simulink model "MovingAvg3"  (R2024b)
settings: Solver=FixedStepAuto  StartTime=0.0  StopTime=1500  FixedStep=1/3600  RelTol=1e-3
undefined symbols (not defined in the file or in its folder): sigbuilder_block
libraries: dspspect3 x1
settings Model: SimulationMode=accelerator  Creator=rupak  LastModifiedBy=rupak
settings ModelReferenceCC: EnableRefExpFcnMdlSchedulingChecks=on
settings RTWCC: GPUComputeCapability=3.5
settings ConfigComp: DVTestSuiteOptimization=Auto  DVDefectChecker=off  DVDetectOutOfBounds=on  DVModelReferenceHarness=on  DVHarnessSource=Signal Editor

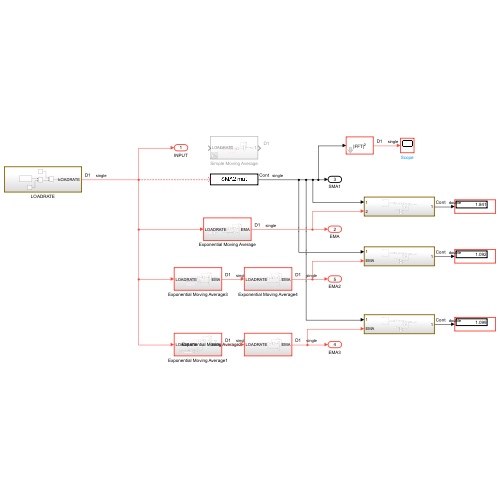
[thumbnail: Simulink's stored preview of the top-level diagram]
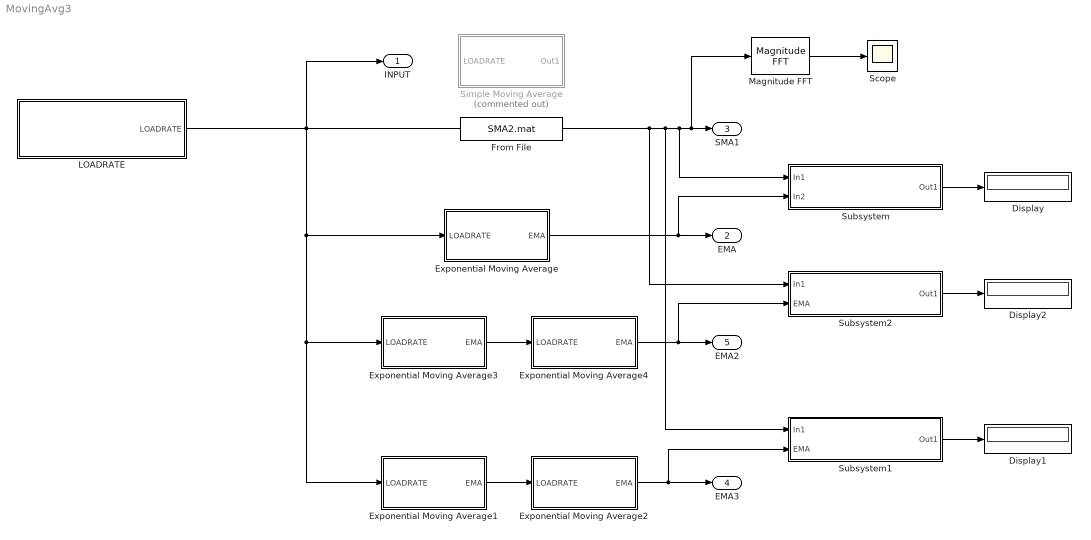
== system MovingAvg3 ==
  Display : Display
  Display1 : Display
  Display2 : Display
  Exponential Moving Average : Subsystem
  Exponential Moving Average1 : Subsystem
  Exponential Moving Average2 : Subsystem
  Exponential Moving Average3 : Subsystem
  Exponential Moving Average4 : Subsystem
  From File : FromFile  FileName=SMA2.mat  SampleTime=0
  LOADRATE : Subsystem
  Magnitude FFT : dspspect3/Magnitude FFT  mag_or_magsq=Magnitude squared  FFTImplementation=Auto  fftLenInherit=off  fftsize=256  WrapInput=on
      settings: LibrarySourceBlock=|
      | dspxfrm3/Magnitude
      | FFT
  Scope : Scope
  Simple Moving Average : Subsystem  Commented=on
  Subsystem : Subsystem
  Subsystem1 : Subsystem
  Subsystem2 : Subsystem
  INPUT : Outport
  EMA : Outport  Port=2
  SMA1 : Outport  Port=3
  EMA3 : Outport  Port=4
  EMA2 : Outport  Port=5
  wires:
  Exponential Moving Average/1(EMA) -> EMA/1, Subsystem/2(In2)
  From File/1 -> Subsystem2/1(In1), Subsystem1/1(In1), Subsystem/1(In1), Magnitude FFT/1, SMA1/1
  Exponential Moving Average1/1(EMA) -> Exponential Moving Average2/1(LOADRATE)
  Exponential Moving Average2/1(EMA) -> EMA3/1, Subsystem1/2(EMA)
  LOADRATE/1(LOADRATE) -> Exponential Moving Average3/1(LOADRATE), Exponential Moving Average1/1(LOADRATE), Exponential Moving Average/1(LOADRATE), INPUT/1
  Subsystem/1(Out1) -> Display/1
  Subsystem1/1(Out1) -> Display1/1
  Exponential Moving Average3/1(EMA) -> Exponential Moving Average4/1(LOADRATE)
  Exponential Moving Average4/1(EMA) -> Subsystem2/2(EMA), EMA2/1
  Subsystem2/1(Out1) -> Display2/1
  Magnitude FFT/1 -> Scope/1

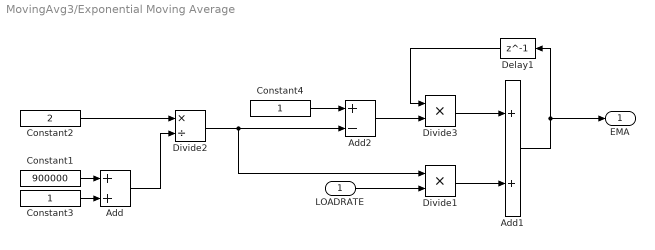
== system MovingAvg3/Exponential Moving Average ==
  LOADRATE : Inport
  Add : Sum
  Add1 : Sum
  Add2 : Sum  Inputs=+-
  Constant1 : Constant  Value=900000  OutDataTypeStr=single
  Constant2 : Constant  Value=2  OutDataTypeStr=single
  Constant3 : Constant  OutDataTypeStr=single
  Constant4 : Constant  OutDataTypeStr=single
  Delay1 : Delay  DelayLength=1  InitialCondition=60
  Divide1 : Product  Inputs=**
  Divide2 : Product  Inputs=*/
  Divide3 : Product  Inputs=**
  EMA : Outport
  wires:
  Add1/1 -> EMA/1, Delay1/1
  Divide1/1 -> Add1/2
  Constant2/1 -> Divide2/1
  Constant1/1 -> Add/1
  Constant3/1 -> Add/2
  Add/1 -> Divide2/2
  Delay1/1 -> Divide3/1
  Divide3/1 -> Add1/1
  Add2/1 -> Divide3/2
  Constant4/1 -> Add2/1
  Divide2/1 -> Add2/2, Divide1/1
  LOADRATE/1 -> Divide1/2

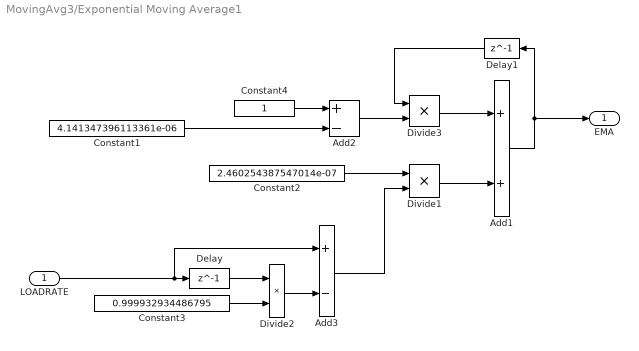
== system MovingAvg3/Exponential Moving Average1 ==
  LOADRATE : Inport
  Add1 : Sum
  Add2 : Sum  Inputs=+-
  Add3 : Sum  Inputs=+-
  Constant1 : Constant  Value=4.141347396113361e-06  OutDataTypeStr=single
  Constant2 : Constant  Value=2.460254387547014e-07  OutDataTypeStr=single
  Constant3 : Constant  Value=0.999932934486795  OutDataTypeStr=single
  Constant4 : Constant  OutDataTypeStr=single
  Delay : Delay  DelayLength=1  InitialCondition=60
  Delay1 : Delay  DelayLength=1  InitialCondition=0.000238234
  Divide1 : Product  Inputs=**
  Divide2 : Product  Inputs=**
  Divide3 : Product  Inputs=**
  EMA : Outport
  wires:
  Add1/1 -> EMA/1, Delay1/1
  Divide1/1 -> Add1/2
  Delay1/1 -> Divide3/1
  Divide3/1 -> Add1/1
  Add2/1 -> Divide3/2
  Constant4/1 -> Add2/1
  Constant1/1 -> Add2/2
  LOADRATE/1 -> Add3/1, Delay/1
  Delay/1 -> Divide2/1
  Constant3/1 -> Divide2/2
  Add3/1 -> Divide1/2
  Divide2/1 -> Add3/2
  Constant2/1 -> Divide1/1

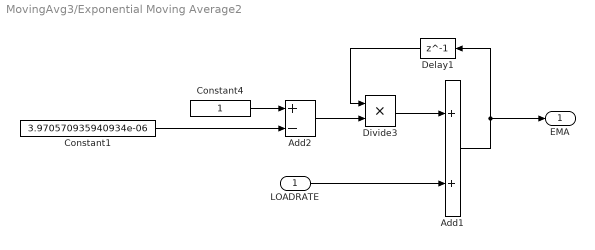
== system MovingAvg3/Exponential Moving Average2 ==
  LOADRATE : Inport
  Add1 : Sum
  Add2 : Sum  Inputs=+-
  Constant1 : Constant  Value=3.970570935940934e-06  OutDataTypeStr=single
  Constant4 : Constant  OutDataTypeStr=single
  Delay1 : Delay  DelayLength=1  InitialCondition=60
  Divide3 : Product  Inputs=**
  EMA : Outport
  wires:
  Add1/1 -> EMA/1, Delay1/1
  LOADRATE/1 -> Add1/2
  Delay1/1 -> Divide3/1
  Divide3/1 -> Add1/1
  Add2/1 -> Divide3/2
  Constant4/1 -> Add2/1
  Constant1/1 -> Add2/2

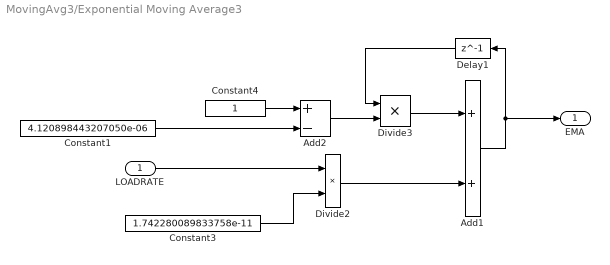
== system MovingAvg3/Exponential Moving Average3 ==
  LOADRATE : Inport
  Add1 : Sum
  Add2 : Sum  Inputs=+-
  Constant1 : Constant  Value=4.120898443207050e-06  OutDataTypeStr=single
  Constant3 : Constant  Value=1.742280089833758e-11  OutDataTypeStr=single
  Constant4 : Constant  OutDataTypeStr=single
  Delay1 : Delay  DelayLength=1  InitialCondition=0.000252816
  Divide2 : Product  Inputs=**
  Divide3 : Product  Inputs=**
  EMA : Outport
  wires:
  Add1/1 -> EMA/1, Delay1/1
  Divide2/1 -> Add1/2
  Delay1/1 -> Divide3/1
  Divide3/1 -> Add1/1
  Add2/1 -> Divide3/2
  Constant4/1 -> Add2/1
  Constant1/1 -> Add2/2
  LOADRATE/1 -> Divide2/1
  Constant3/1 -> Divide2/2

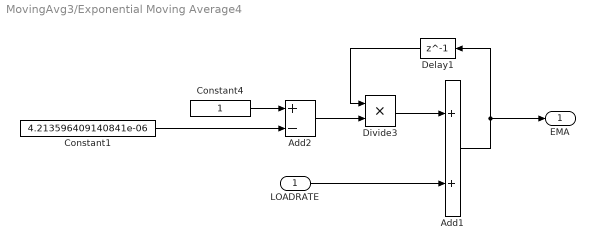
== system MovingAvg3/Exponential Moving Average4 ==
  LOADRATE : Inport
  Add1 : Sum
  Add2 : Sum  Inputs=+-
  Constant1 : Constant  Value=4.213596409140841e-06  OutDataTypeStr=single
  Constant4 : Constant  OutDataTypeStr=single
  Delay1 : Delay  DelayLength=1  InitialCondition=60
  Divide3 : Product  Inputs=**
  EMA : Outport
  wires:
  Add1/1 -> EMA/1, Delay1/1
  LOADRATE/1 -> Add1/2
  Delay1/1 -> Divide3/1
  Divide3/1 -> Add1/1
  Add2/1 -> Divide3/2
  Constant4/1 -> Add2/1
  Constant1/1 -> Add2/2

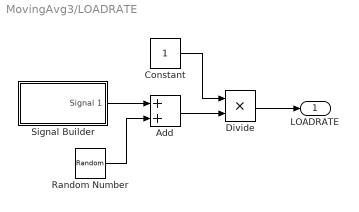
== system MovingAvg3/LOADRATE ==
  Add : Sum
  Constant : Constant  OutDataTypeStr=single
  Divide : Product  Inputs=**  OutDataTypeStr=Inherit: Same as first input
  Random Number : RandomNumber  Mean=5  SampleTime=1/3600
  Signal Builder : Subsystem  Tag=STV Subsys  LoadFcn=sigbuilder_block('load');  StartFcn=sigbuilder_block('start');  StopFcn=sigbuilder_block('stop');  ClipboardFcn=sigbuilder_block('clipboard');  mask(Sigbuilder block){tuvar=[0:10]}
      mask help: Simulink:masks:SigbuilderBlock_MD
      mask init:
      | if ~strcmp(get_param(bdroot(gcbh),'SimulationStatus'),'stopped') tuvar = sigbuilder_block('maskInit'); end
      settings: CopyFcn=sigbuilder_block('copy');  DeleteFcn=sigbuilder_block('delete');  ModelCloseFcn=sigbuilder_block('modelClose');  PreSaveFcn=sigbuilder_block('preSave');  PauseFcn=sigbuilder_block('pause');  ContinueFcn=sigbuilder_block('continue');  NameChangeFcn=sigbuilder_block('namechange');  OpenFcn=sigbuilder_block('open',[6 36 1428 675.75 ]);  CloseFcn=sigbuilder_block('close');
      mask Display: plot(0, 0, 100, 100,[2, 2, 32, 32, 2], [68, 8, 8, 68, 68],[32, 2], [38, 38], [32, 19, 2],[53, 60, 44], [32, 17, 17, 2],[16, 16, 31, 31]);txt = getActiveGroup(gcbh);text(2, 100, txt,'verticalAlignment', 'top');
  LOADRATE : Outport  SampleTime=1/3600
  wires:
  Random Number/1 -> Add/2
  Signal Builder/1(Signal 1) -> Add/1
  Add/1 -> Divide/2
  Divide/1 -> LOADRATE/1
  Constant/1 -> Divide/1

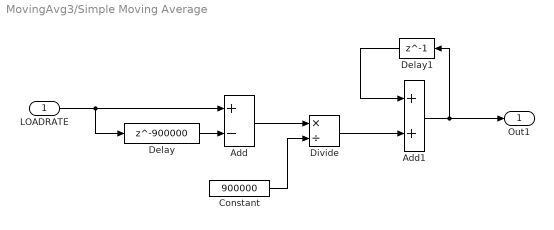
== system MovingAvg3/Simple Moving Average ==
  LOADRATE : Inport
  Add : Sum  Inputs=+-
  Add1 : Sum
  Constant : Constant  Value=900000  OutDataTypeStr=single
  Delay : Delay  DelayLength=900000  InitialCondition=60
  Delay1 : Delay  DelayLength=1  InitialCondition=60
  Divide : Product  Inputs=*/
  Out1 : Outport
  wires:
  Delay/1 -> Add/2
  Delay1/1 -> Add1/1
  Constant/1 -> Divide/2
  LOADRATE/1 -> Delay/1, Add/1
  Add/1 -> Divide/1
  Add1/1 -> Out1/1, Delay1/1
  Divide/1 -> Add1/2

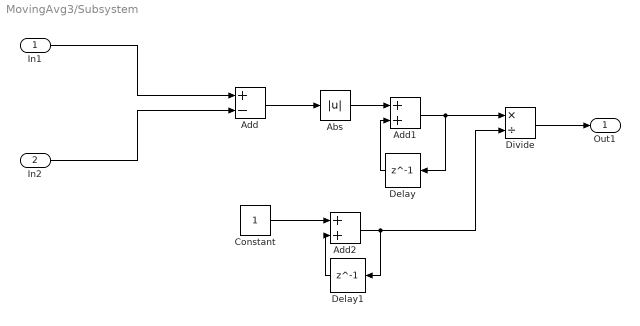
== system MovingAvg3/Subsystem ==
  In1 : Inport
  In2 : Inport  Port=2
  Abs : Abs  SaturateOnIntegerOverflow=off
  Add : Sum  Inputs=+-
  Add1 : Sum
  Add2 : Sum
  Constant : Constant
  Delay : Delay  DelayLength=1
  Delay1 : Delay  DelayLength=1
  Divide : Product  Inputs=*/
  Out1 : Outport
  wires:
  Add/1 -> Abs/1
  Add2/1 -> Divide/2, Delay1/1
  Delay1/1 -> Add2/2
  In1/1 -> Add/1
  Add1/1 -> Delay/1, Divide/1
  Delay/1 -> Add1/2
  In2/1 -> Add/2
  Abs/1 -> Add1/1
  Constant/1 -> Add2/1
  Divide/1 -> Out1/1

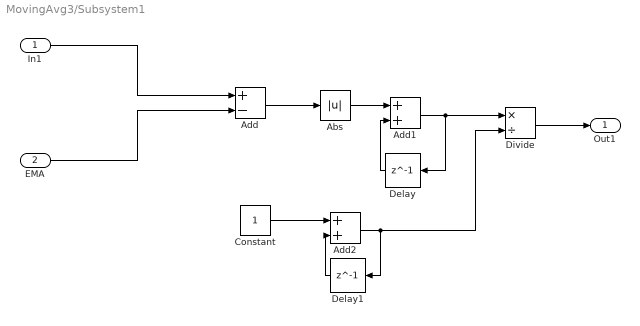
== system MovingAvg3/Subsystem1 ==
  In1 : Inport
  EMA : Inport  Port=2
  Abs : Abs  SaturateOnIntegerOverflow=off
  Add : Sum  Inputs=+-
  Add1 : Sum
  Add2 : Sum
  Constant : Constant
  Delay : Delay  DelayLength=1
  Delay1 : Delay  DelayLength=1
  Divide : Product  Inputs=*/
  Out1 : Outport
  wires:
  Divide/1 -> Out1/1
  Constant/1 -> Add2/1
  Abs/1 -> Add1/1
  EMA/1 -> Add/2
  Delay/1 -> Add1/2
  Add1/1 -> Divide/1, Delay/1
  In1/1 -> Add/1
  Delay1/1 -> Add2/2
  Add2/1 -> Delay1/1, Divide/2
  Add/1 -> Abs/1

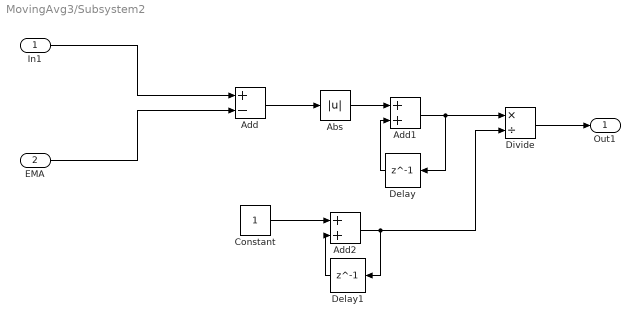
== system MovingAvg3/Subsystem2 ==
  In1 : Inport
  EMA : Inport  Port=2
  Abs : Abs  SaturateOnIntegerOverflow=off
  Add : Sum  Inputs=+-
  Add1 : Sum
  Add2 : Sum
  Constant : Constant
  Delay : Delay  DelayLength=1
  Delay1 : Delay  DelayLength=1
  Divide : Product  Inputs=*/
  Out1 : Outport
  wires:
  Divide/1 -> Out1/1
  Constant/1 -> Add2/1
  Abs/1 -> Add1/1
  EMA/1 -> Add/2
  Delay/1 -> Add1/2
  Add1/1 -> Divide/1, Delay/1
  In1/1 -> Add/1
  Delay1/1 -> Add2/2
  Add2/1 -> Delay1/1, Divide/2
  Add/1 -> Abs/1

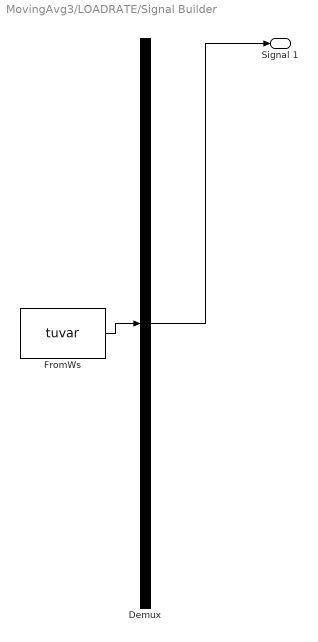
== system MovingAvg3/LOADRATE/Signal Builder ==
  Demux : Demux  Tag=STV Demux  Outputs=1
      settings: DisplayOption=none
  FromWs : FromWorkspace  Tag=STV FromWs  VariableName=tuvar
      SigBuilderData=|
      | common.afterFinalStr = 'Extrapolate'
      | common.sampleTime = 0
      | dataSet.timeRange = [0 1500]
      | dataSet.name = 'Group 1'
      | sbobj.Groups.Name = 'Group 1'
      | sbobj.Groups.Signals.Name = 'Signal 1'
      | sbobj.Groups.Signals.XData = [0 4 4 10 12 16 18 20 24 30 36 40 44 50 56 60 60 64 64 70 74 78 80 82 86 88 88 90 92 98 104 108 112 118 122 128 132 138 144 150 154 158 160 162 166 170 174 176 180 182 184 190 196 200 202 208 216 226 232 240 250 260 266 278 284 292 296 300 304 310 316 322 326 338 346 356 362 368 374 378 384 392 400 406 414 420 424 430 432 438 442 446 450 458 464 470 476 482 487 489 490 496 500 508 518 528 536 546 552 558 562 570 582 588 592 598 606 620 626 634 644 650 664 673 674 682 696 706 716 724 734 744 756 764 772 780 790 800 808 816 826 834 844 856 864 872 880 890 904 914 928 942 952 960 972 994 1072 1116 1126 1134 1142 1156 1160 1166 1176 1182 1190 1198 1208 1220 1228 1235 1246 1258 1265 1277 1287 1297 1308 1323 1332 1342 1347 1355 1361 1371 1379 1389 1402 1408 1415 1422 1435 1439 1446 1453 1469 1475 1485 1492 1495 1500]
      | sbobj.Groups.Signals.YData = [2 96.2 69.2 84 75 56.8 90 74.4 80.8 65.2 91 85.4 67.4 77.4 55.6 61 48 18.6 31.6 51.4 51.4 38.4 56.4 63.4 86.6 78.2 83.2 71 57.6 78.6 36 85.4 57 39 41 43.8 57 45.6 42.8 53 78.2 68.4 74 67 56.6 61 55.6 34 51.4 74.2 50.8 93 74.4 78 61.2 52 58 40.6 58 54.4 42.6 71 47.8 56 50.8 69 48.2 70 54.8 48.2 54.6 34.4 46.4 55.6 42.6 57.2 33.2 85.8 53.6 59 54.6 49.4 63 54.8 76.4 57.2 70 64.8 35.4 64.2 51.8 57 47.2 59.8 52.6 69 53.4 70 64.8 61.4 45.4 53.4 32 46.8 42.6 45 39.8 53.6 50.2 59.2 56.8 55 62.2 53.6 56 58.8 56 63 55 66 59.6 71 67.8 70.8 63.4 58 63.2 60.2 63 74.8 63.8 68 59.8 65.6 55.6 63.2 62.2 68.6 65.6 69.6 69 75.2 70 72 66.6 63.4 86 74.4 83.4 79 61.6 69.8 51.2 60.4 40.4 49.6 33 40.6 45.8 43.4 49.8 45 48.8 55 49.6 44.4 56 52 67 55 52 56.6 48.6 57 52.4 62.2 46.8 59.2 60.6 57.4 65.2 63.2238095238 66.2 76.2 70 75 82.2 72.2 75.4 69.4 72.4 65.2 66.2 64.0953846154 65.6 65.4 65.4 59.8 59.6 63.2 57.2 51.4]
      | sbobj.Groups.TimeRange = [0 1500]
  Signal 1 : Outport  Tag=STV Outport
  wires:
  Demux/1 -> Signal 1/1
  FromWs/1 -> Demux/1
